simulink model "feedback_integrator"  (R2017a)
settings: Solver=VariableStepAuto  StartTime=0.0  StopTime=10  RelTol=1e-3
values from neighbouring files (symbols this model uses):
  A = [0 1;0 0]    [Adaptive_Control.m]    (also in Adaptive_Control_Linear.m = [0 1;a1 a2]; HGO.m = [0 1;-1 -1]; Non_linear_observers_.m; feedback-integrator.m = [1 1;0 0])
  B = [0;1]    [Adaptive_Control.m]    (also in Adaptive_Control_Linear.m = [0;b]; Non_linear_observers_.m; feedback-integrator.m = [0;1+b]; mini_projet.m = [0;1+b])
  ki = Kaug(3)    [Adaptive_Control_Linear.m]    (also in mini_projet.m = kk(3))
  kp = [kk(1) kk(2)]    [mini_projet.m]
settings Model: Creator=firass2019  LastModifiedBy=firass2019

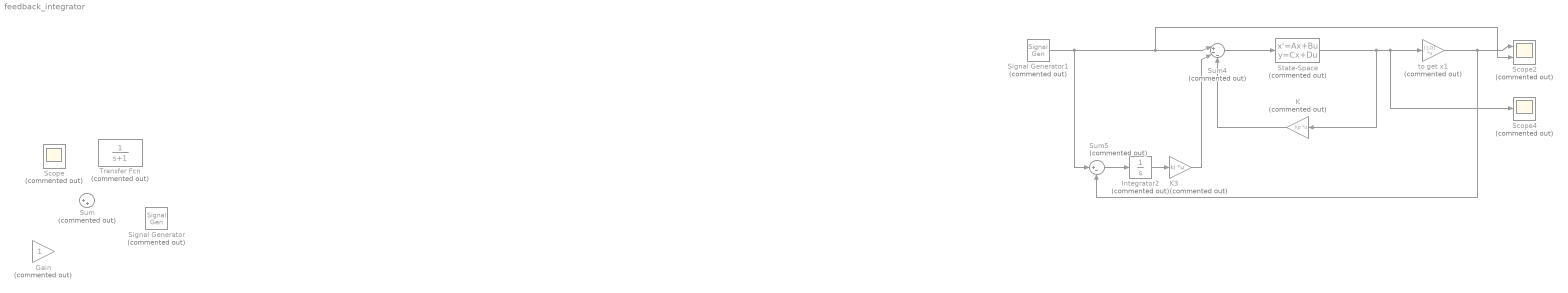
== system feedback_integrator ==
  Gain : Gain  Commented=on
  Integrator2 : Integrator  Commented=on
  K : Gain  Commented=on  Gain=kp  Multiplication=Matrix(K*u)
  K3 : Gain  Commented=on  Gain=ki  Multiplication=Matrix(K*u)
  Scope : Scope  Commented=on
  Scope2 : Scope  Commented=on  NumInputPorts=2
  Scope4 : Scope  Commented=on
  Signal Generator : SignalGenerator  Commented=on  Units=rad/sec
  Signal Generator1 : SignalGenerator  Commented=on  WaveForm=square  Units=rad/sec
  State-Space : StateSpace  Commented=on  A=A  B=B  C=[1,0;0 1]  D=[0;0]  X0=0
  Sum : Sum  Commented=on  Inputs=|++
  Sum4 : Sum  Commented=on  Inputs=|+--
  Sum5 : Sum  Commented=on  Inputs=|+-
  Transfer Fcn : TransferFcn  Commented=on  Denominator=[1 1]
  to get x1 : Gain  Commented=on  Gain=[1,0]  Multiplication=Matrix(K*u)
  wires:
  State-Space/1 -> Scope4/1, to get x1/1, K/1
  Signal Generator1/1 -> Scope2/2, Sum4/1, Sum5/1
  Sum4/1 -> State-Space/1
  to get x1/1 -> Sum5/2, Scope2/1
  Sum5/1 -> Integrator2/1
  Integrator2/1 -> K3/1
  K/1 -> Sum4/3
  K3/1 -> Sum4/2
